simulink model "PD"  (R2020a)
settings: Solver=FixedStepAuto  StartTime=0.0  StopTime=200  RelTol=1e-3  EnableMultiTasking=on
values from neighbouring files (symbols this model uses):
  down = -up    (= -0.0872664625997)    [PD_statespace.m]
  Kx = place(A_d_x,1.1*B_d_x,p_d_x)    [PD_statespace.m]
  Ky = place(A_d_y,1.1*B_d_y,p_d_y)    [PD_statespace.m]
  Ts = 0.02    [PD_statespace.m]
  up = 5*pi/180    (= 0.0872664625997)    [PD_statespace.m]
undefined symbols (not defined in the file or in its folder): A_d_x, A_d_y, B_d_x, B_d_y, C_d_x, C_d_y, DiscIntNeverNeededParam
libraries: raspberrypiBasiclib x6, simulink x4, raspberrypiCommlib x1
settings Model: Creator=hhiastt  LastModifiedBy=hhiastt
settings SolverCC: PositivePriorityOrder=on
settings OptimizationCC: EnhancedBackFolding=on  PassReuseOutputArgsAs=Individual arguments  ZeroExternalMemoryAtStartup=off  ZeroInternalMemoryAtStartup=off  MaxStackSize=64  OptimizeBlockOrder=speed  DifferentSizesBufferReuse=on  OptimizationCustomize=off  EfficientTunableParamExpr=on
settings DebuggingCC: ParameterTunabilityLossMsg=error
settings HardwareCC: ProdBitPerPointer=32  ProdBitPerSizeT=32  ProdBitPerPtrDiffT=32  ProdLargestAtomicInteger=Long  ProdLargestAtomicFloat=Double  ProdWordSize=32  ProdLongLongMode=on  ProdHWDeviceType=ARM Compatible->ARM Cortex
settings RTWCC: SystemTargetFile=ert.tlc  HardwareBoard=Raspberry Pi  TemplateMakefile=ert_default_tmf  Toolchain=GNU GCC Raspberry Pi  BuildConfiguration=Faster Runs
settings CodeAppCC: ForceParamTrailComments=on  IgnoreCustomStorageClasses=off  OperatorAnnotations=on  SimulinkDataObjDesc=on  SFDataObjDesc=on  InsertBlockDesc=on
settings ERTTargetCC: SupportVariableSizeSignals=on

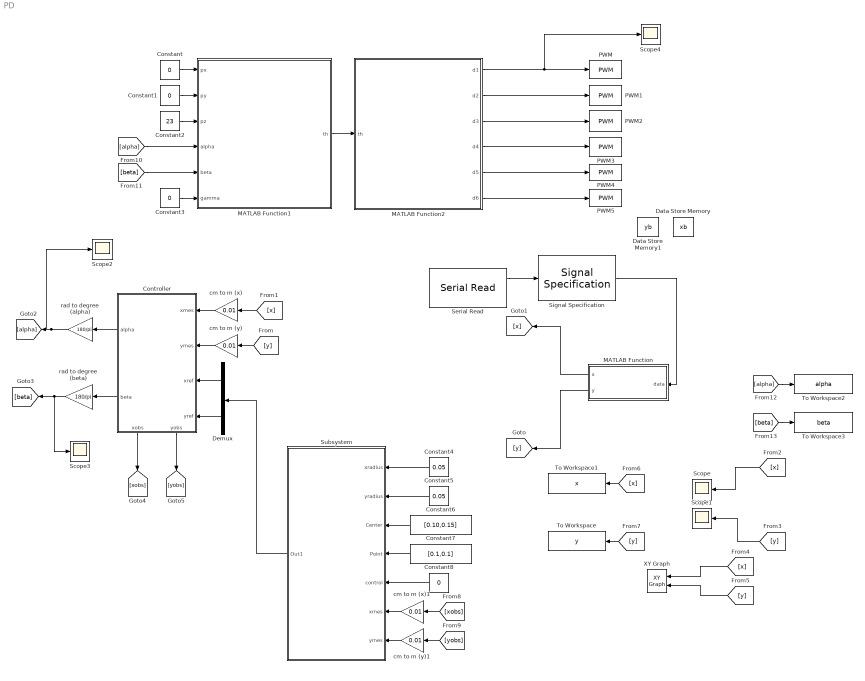
== system PD ==
  Constant{,1,3,8} (4 alike) : Constant  Value=0
  Constant2 : Constant  Value=23
  Constant4 : Constant  Value=0.05
  Constant5 : Constant  Value=0.05
  Constant6 : Constant  Value=[0.10,0.15]
  Constant7 : Constant  Value=[0.1,0.1]
  Controller : Subsystem
      settings: PortSchema="{\"entries\":[{\"content\":{\"sides\":[{\"content\":{\"connectorIds\":[\"In1\",\"In2\",\"In3\",\"In4\"]},\"type\":\"ConnectorPlacement.EquallySpacedRectSide\",\"uuid\":\"b3f4a7cd-8500-437d-beb5-3714d996e55f\"},{\"content\":{\"connectorIds\":[\"Out1\",\"Out2\"],\"side\":\"RIGHT\"},\"type\":\"ConnectorPlacement.EquallySpacedRectSide\",\"uuid\":\"7399a696-fe70-41e1-908f-e26d67b443d7\"},{\"content\":{\"connectorIds\":[],\"side\":\"TOP\"},\"type\":\"ConnectorPlacement.EquallySpacedRectSide\",\"uuid\":\"0bf1a723-c9e2-46e2-b0a4-128eb8cfe212\"},{\"content\":{\"connectorIds\":[\"Out3\",\"Out4\"],\"side\":\"BOTTOM\"},\"type\":\"ConnectorPlacement.EquallySpacedRectSide\",\"uuid\":\"22262538-2ead-478c-9765-503d5c54f33f\"}]},\"type\":\"ConnectorPlacement.EquallySpacedConnector\",\"uuid\":\"64fddb79-6683-4736-8f96-8b1913bbda93\"}],\"packageUris\":[\"http://schema.mathworks.com/mf0/Connector/19700101\"],\"version\":\"1.0\"}"
  Data Store Memory : DataStoreMemory  DataStoreName=xb  ReadBeforeWriteMsg=warning  WriteAfterWriteMsg=warning  WriteAfterReadMsg=warning  ShowAdditionalParam=off  OutDataTypeStr=double
  Data Store Memory1 : DataStoreMemory  DataStoreName=yb  ReadBeforeWriteMsg=warning  WriteAfterWriteMsg=warning  WriteAfterReadMsg=warning  ShowAdditionalParam=off  OutDataTypeStr=double
  Demux : Demux  Outputs=2
  MATLAB Function : MATLAB Function  TreatAsAtomicUnit=on
  MATLAB Function1 : MATLAB Function  TreatAsAtomicUnit=on
  MATLAB Function2 : MATLAB Function  TreatAsAtomicUnit=on
  PWM : raspberrypiBasiclib/PWM  board=Pi 3 Model B+  Pin_=12  Frequency=50  blockPlatform=Raspberry Pi
      settings: SourceProductBaseCode=RASPPI
  PWM1 : raspberrypiBasiclib/PWM  board=Pi 3 Model B+  Pin_=20  Frequency=50  blockPlatform=Raspberry Pi
      settings: SourceProductBaseCode=RASPPI
  PWM2 : raspberrypiBasiclib/PWM  board=Pi 3 Model B+  Pin_=26  Frequency=50  blockPlatform=Raspberry Pi
      settings: SourceProductBaseCode=RASPPI
  PWM3 : raspberrypiBasiclib/PWM  board=Pi 3 Model B+  Pin_=17  Frequency=50  blockPlatform=Raspberry Pi
      settings: SourceProductBaseCode=RASPPI
  PWM4 : raspberrypiBasiclib/PWM  board=Pi 3 Model B+  Pin_=27  Frequency=50  blockPlatform=Raspberry Pi
      settings: SourceProductBaseCode=RASPPI
  PWM5 : raspberrypiBasiclib/PWM  board=Pi 3 Model B+  Pin_=22  Frequency=50  blockPlatform=Raspberry Pi
      settings: SourceProductBaseCode=RASPPI
  Scope{,1..4} (5 alike) : Scope
  Serial Read : raspberrypiCommlib/Serial Read  board=Pi 3 Model B+  SCIModule_=/dev/ttyS0  Baudrate_=19200  Parity=None  StopBits_=1  HardwareFlowControl=None  ByteOrder=LittleEndian  DataLength=10  DataType=uint8  OutputStatus=on  SampleTime=Ts  blockPlatform=RaspberryPi
      settings: SourceProductBaseCode=RASPPI
  Signal Specification : SignalSpecification  OutDataTypeStr=uint8  Dimensions=10  SampleTime=Ts
  Subsystem : Subsystem
  To Workspace : ToWorkspace  VariableName=y  SampleTime=Ts
      settings: Save2DSignal=2-D array (concatenate along first dimension)
  To Workspace1 : ToWorkspace  VariableName=x  SampleTime=Ts
      settings: Save2DSignal=2-D array (concatenate along first dimension)
  To Workspace2 : ToWorkspace  VariableName=alpha  SaveFormat=Timeseries  SampleTime=-1
  To Workspace3 : ToWorkspace  VariableName=beta  SaveFormat=Timeseries  SampleTime=-1
  XY Graph : simulink/Sinks/XY Graph  xmin=0  xmax=20  ymin=0  ymax=30  st=Ts
  cm to m (x) : Gain  Gain=0.01
  cm to m (x)1 : Gain  Gain=0.01
  cm to m (y) : Gain  Gain=0.01
  cm to m (y)1 : Gain  Gain=0.01
  rad to degree (alpha) : Gain  Gain=180/pi
  rad to degree (beta) : Gain  Gain=180/pi
  wires:
  Constant2/1 -> MATLAB Function1/3(pz)
  [x] -> cm to m (x)/1
  MATLAB Function2/5(d5) -> PWM4/1
  Constant8/1 -> Subsystem/5(control)
  rad to degree (beta)/1 -> Scope3/1, [beta]
  [y] -> cm to m (y)/1
  cm to m (x)1/1 -> Subsystem/6(xmes)
  Controller/1(alpha) -> rad to degree (alpha)/1
  Controller/2(beta) -> rad to degree (beta)/1
  Demux/1 -> Controller/3(xref)
  [yobs] -> cm to m (y)1/1
  cm to m (y)/1 -> Controller/2(ymes)
  rad to degree (alpha)/1 -> Scope2/1, [alpha]
  Constant6/1 -> Subsystem/3(Center)
  Constant5/1 -> Subsystem/2(yradius)
  [x] -> To Workspace1/1
  Constant4/1 -> Subsystem/1(xradius)
  [alpha] -> MATLAB Function1/4(alpha)
  [y] -> XY Graph/2
  cm to m (y)1/1 -> Subsystem/7(ymes)
  Constant3/1 -> MATLAB Function1/6(gamma)
  [xobs] -> cm to m (x)1/1
  Constant/1 -> MATLAB Function1/1(px)
  cm to m (x)/1 -> Controller/1(xmes)
  [beta] -> MATLAB Function1/5(beta)
  MATLAB Function2/6(d6) -> PWM5/1
  Signal Specification/1 -> MATLAB Function/1(data)
  MATLAB Function1/1(th) -> MATLAB Function2/1(th)
  [y] -> To Workspace/1
  MATLAB Function/1(x) -> [x]
  MATLAB Function2/2(d2) -> PWM1/1
  [x] -> XY Graph/1
  MATLAB Function2/4(d4) -> PWM3/1
  MATLAB Function2/1(d1) -> Scope4/1, PWM/1
  Constant1/1 -> MATLAB Function1/2(py)
  MATLAB Function/2(y) -> [y]
  Demux/2 -> Controller/4(yref)
  MATLAB Function2/3(d3) -> PWM2/1
  Serial Read/1 -> Signal Specification/1
  Constant7/1 -> Subsystem/4(Point)
  Controller/4(xobs) -> [xobs]
  Controller/3(yobs) -> [yobs]
  Subsystem/1(Out1) -> Demux/1
  [x] -> Scope/1
  [y] -> Scope1/1
  [alpha] -> To Workspace2/1
  [beta] -> To Workspace3/1

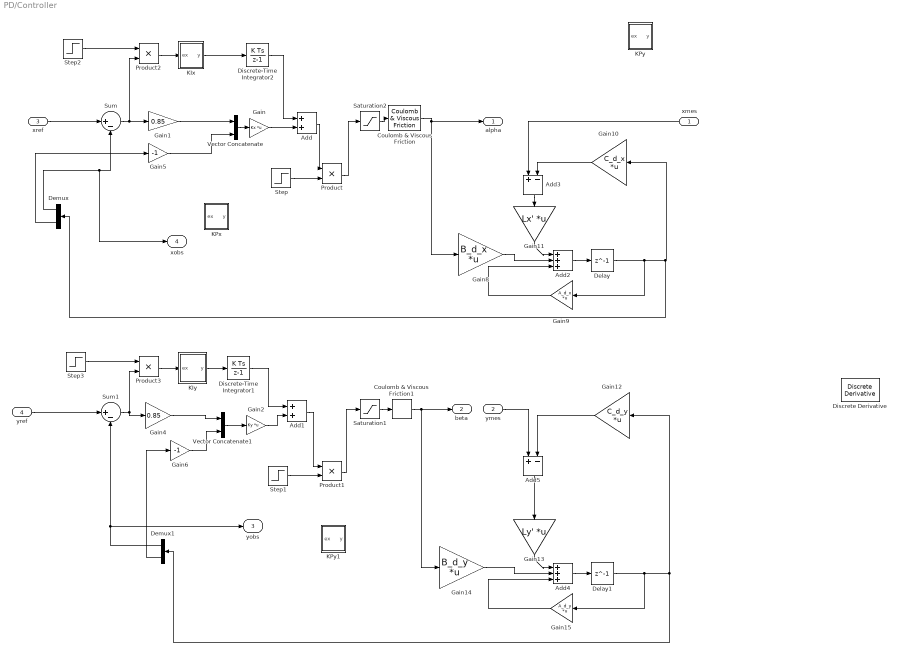
== system PD/Controller ==
  xmes : Inport
  ymes : Inport  Port=2
  xref : Inport  Port=3
  yref : Inport  Port=4
  Add : Sum
  Add1 : Sum
  Add2 : Sum  Inputs=+++
  Add3 : Sum  Inputs=+-
  Add4 : Sum  Inputs=+++
  Add5 : Sum  Inputs=+-
  Coulomb & Viscous Friction : simulink/Discontinuities/Coulomb & Viscous Friction  offset=[0.15*pi/180]  gain=1
  Coulomb & Viscous Friction1 : simulink/Discontinuities/Coulomb & Viscous Friction  offset=[0.15*pi/180]  gain=1
  Delay : Delay  DelayLength=1  SampleTime=Ts
  Delay1 : Delay  DelayLength=1  SampleTime=Ts
  Demux : Demux  Outputs=2
  Demux1 : Demux  Outputs=2
  Discrete Derivative : simulink/Discrete/Discrete Derivative  gainval=1.0  ICPrevScaledInput=0.0  OutMin=[]  OutMax=[]  OutDataType=fixdt(1, 16)  OutScaling=2^-10  DoSatur=off
  Discrete-Time Integrator1 : DiscreteIntegrator  SampleTime=-1  ICPrevOutput=DiscIntNeverNeededParam  ICPrevScaledInput=DiscIntNeverNeededParam
  Discrete-Time Integrator2 : DiscreteIntegrator  SampleTime=-1  ICPrevOutput=DiscIntNeverNeededParam  ICPrevScaledInput=DiscIntNeverNeededParam
  Gain : Gain  Gain=Kx  Multiplication=Matrix(K*u)
  Gain1 : Gain  Gain=0.85
  Gain10 : Gain  Gain=C_d_x  Multiplication=Matrix(K*u)
  Gain11 : Gain  Gain=Lx'  Multiplication=Matrix(K*u)
  Gain12 : Gain  Gain=C_d_y  Multiplication=Matrix(K*u)
  Gain13 : Gain  Gain=Ly'  Multiplication=Matrix(K*u)
  Gain14 : Gain  Gain=B_d_y  Multiplication=Matrix(K*u)
  Gain15 : Gain  Gain=A_d_y  Multiplication=Matrix(K*u)
  Gain2 : Gain  Gain=Ky  Multiplication=Matrix(K*u)
  Gain4 : Gain  Gain=0.85
  Gain5 : Gain  Gain=-1
  Gain6 : Gain  Gain=-1
  Gain8 : Gain  Gain=B_d_x  Multiplication=Matrix(K*u)
  Gain9 : Gain  Gain=A_d_x  Multiplication=Matrix(K*u)
  KIx : MATLAB Function  TreatAsAtomicUnit=on
  KIy : MATLAB Function  TreatAsAtomicUnit=on
  KPx : MATLAB Function  TreatAsAtomicUnit=on
  KPy : MATLAB Function  TreatAsAtomicUnit=on
  KPy1 : MATLAB Function  TreatAsAtomicUnit=on
  Product{,1..3} (4 alike) : Product
  Saturation1 : Saturate  UpperLimit=up  LowerLimit=down
  Saturation2 : Saturate  UpperLimit=up  LowerLimit=down
  Step{,1..3} (4 alike) : Step  Time=4  SampleTime=Ts
  Sum : Sum  Inputs=|+-
  Sum1 : Sum  Inputs=|+-
  Vector Concatenate : Concatenate
  Vector Concatenate1 : Concatenate
  alpha : Outport
  beta : Outport  Port=2
  yobs : Outport  Port=3
  xobs : Outport  Port=4
  wires:
  xref/1 -> Sum/1
  yref/1 -> Sum1/1
  Demux1/2 -> Gain6/1
  Saturation2/1 -> Coulomb & Viscous Friction/1
  xmes/1 -> Add3/1
  Gain9/1 -> Add2/3
  Gain8/1 -> Add2/2
  Gain11/1 -> Add2/1
  Delay/1 -> Demux/1, Gain10/1, Gain9/1
  Add3/1 -> Gain11/1
  Gain10/1 -> Add3/2
  Add2/1 -> Delay/1
  ymes/1 -> Add5/1
  Demux1/1 -> yobs/1, Sum1/2
  Add4/1 -> Delay1/1
  Gain13/1 -> Add4/1
  Add5/1 -> Gain13/1
  Delay1/1 -> Gain15/1, Demux1/1, Gain12/1
  Gain12/1 -> Add5/2
  Gain14/1 -> Add4/2
  Gain15/1 -> Add4/3
  Demux/1 -> xobs/1, Sum/2
  Sum/1 -> Gain1/1, Product2/2
  Demux/2 -> Gain5/1
  Sum1/1 -> Gain4/1, Product3/2
  KIx/1(y) -> Discrete-Time Integrator2/1
  KIy/1(y) -> Discrete-Time Integrator1/1
  Step/1 -> Product/2
  Step1/1 -> Product1/2
  Add/1 -> Product/1
  Product/1 -> Saturation2/1
  Add1/1 -> Product1/1
  Product1/1 -> Saturation1/1
  Step2/1 -> Product2/1
  Product2/1 -> KIx/1(ex)
  Product3/1 -> KIy/1(ex)
  Step3/1 -> Product3/1
  Gain5/1 -> Vector Concatenate/2
  Vector Concatenate/1 -> Gain/1
  Gain/1 -> Add/2
  Vector Concatenate1/1 -> Gain2/1
  Gain6/1 -> Vector Concatenate1/2
  Gain2/1 -> Add1/2
  Gain1/1 -> Vector Concatenate/1
  Gain4/1 -> Vector Concatenate1/1
  Discrete-Time Integrator2/1 -> Add/1
  Discrete-Time Integrator1/1 -> Add1/1
  Coulomb & Viscous Friction/1 -> alpha/1, Gain8/1
  Saturation1/1 -> Coulomb & Viscous Friction1/1
  Coulomb & Viscous Friction1/1 -> beta/1, Gain14/1

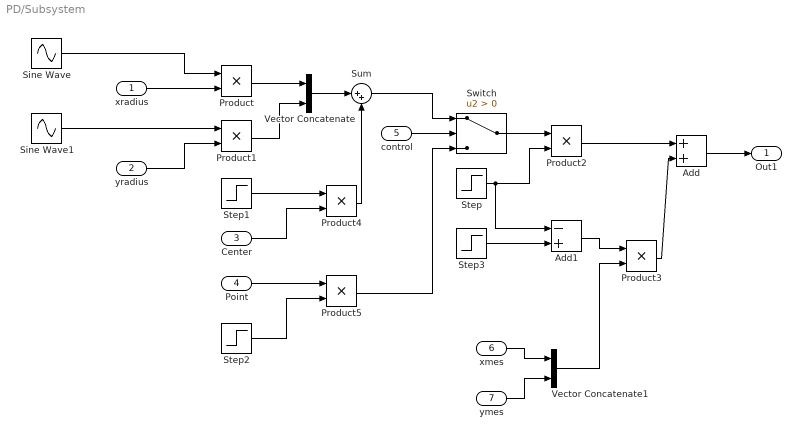
== system PD/Subsystem ==
  xradius : Inport
  yradius : Inport  Port=2
  Center : Inport  Port=3
  Point : Inport  Port=4
  control : Inport  Port=5
  xmes : Inport  Port=6
  ymes : Inport  Port=7
  Add : Sum
  Add1 : Sum  Inputs=-+
  Product{,1..5} (6 alike) : Product
  Sine Wave : Sin  Frequency=0.5  SampleTime=Ts
  Sine Wave1 : Sin  Frequency=0.5  Phase=pi/2  SampleTime=Ts
  Step : Step  Time=4  SampleTime=Ts
  Step1 : Step  Time=0  SampleTime=Ts
  Step2 : Step  Time=0  SampleTime=Ts
  Step3 : Step  Time=0  SampleTime=Ts
  Sum : Sum  Inputs=|++
  Switch : Switch  Criteria=u2 > Threshold
  Vector Concatenate : Concatenate
  Vector Concatenate1 : Concatenate
  Out1 : Outport
  wires:
  Sine Wave/1 -> Product/1
  Sine Wave1/1 -> Product1/1
  xradius/1 -> Product/2
  yradius/1 -> Product1/2
  Product/1 -> Vector Concatenate/1
  Product1/1 -> Vector Concatenate/2
  Vector Concatenate/1 -> Sum/1
  control/1 -> Switch/2
  Sum/1 -> Switch/1
  Product2/1 -> Add/1
  xmes/1 -> Vector Concatenate1/1
  ymes/1 -> Vector Concatenate1/2
  Vector Concatenate1/1 -> Product3/2
  Product3/1 -> Add/2
  Add/1 -> Out1/1
  Switch/1 -> Product2/1
  Step/1 -> Add1/1, Product2/2
  Add1/1 -> Product3/1
  Step1/1 -> Product4/1
  Center/1 -> Product4/2
  Product4/1 -> Sum/2
  Point/1 -> Product5/1
  Product5/1 -> Switch/3
  Step2/1 -> Product5/2
  Step3/1 -> Add1/2

== matlab function PD/MATLAB Function1 ==
  data: px input double size=1; th output double; py input double size=1; pz input double size=1; alpha input double size=1; beta input double size=1; gamma input double size=1
function th = inv_ken_test(px,py,pz,alpha,beta,gamma)
th=zeros(1,6);
l1=3.2;
l2=25.57;
b=26;
d=20;
b1=30;
d1=6;
RA1=[(1/sqrt(12))*(2*b+d);d/2;0];
RA2=[-(1/sqrt(12))*(b-d);(b+d)/2;0];
RA3=[-(1/sqrt(12))*(b+2*d);b/2;0];
RA4=[-(1/sqrt(12))*(b+2*d);-b/2;0];
RA5=[-(1/sqrt(12))*(b-d);-(b+d)/2;0];
RA6=[(1/sqrt(12))*(2*b+d);-d/2;0];
RA=[RA1 RA2 RA3 RA4 RA5 RA6];

RC1=[(1/sqrt(12))*(b1+2*d1);b1/2;0];
RC2=[(1/sqrt(12))*(b1-d1);(b1+d1)/2;0];
RC3=[-(1/sqrt(12))*(2*b1+d1);d1/2;0];
RC4=[-(1/sqrt(12))*(2*b1+d1);-d1/2;0];
RC5=[(1/sqrt(12))*(b1-d1);-(b1+d1)/2;0];
RC6=[(1/sqrt(12))*(b1+2*d1);-b1/2;0];
RC=[RC1 RC2 RC3 RC4 RC5 RC6];

v=[0 0 0 1];
T_base_A1=[rotz(150)*rotx(90) RA1;v];
T_base_A2=[rotz(-30)*rotx(90) RA2;v];
T_base_A3=[rotz(-90)*rotx(90) RA3;v];
T_base_A4=[rotz(90)*rotx(90) RA4;v];
T_base_A5=[rotz(30)*rotx(90) RA5;v];
T_base_A6=[rotz(-150)*rotx(90) RA6;v];

% Computation
R=[rotz(gamma)*roty(beta)*rotx(alpha);0 0 0];
P=[px;py;pz;1];
T=[R P];
RCE=T*[RC;ones(1,6)];
RAE=[RA;ones(1,6)];
L=zeros(1,6);
for i =1:6
    L(i)=sum((RCE(:,i)-RAE(:,i)).^2)^0.5;
end

RA1C1=T_base_A1^(-1)*(RCE(:,1)-RAE(:,1));
RA2C2=T_base_A2^(-1)*(RCE(:,2)-RAE(:,2));
RA3C3=T_base_A3^(-1)*(RCE(:,3)-RAE(:,3));
RA4C4=T_base_A4^(-1)*(RCE(:,4)-RAE(:,4));
RA5C5=T_base_A5^(-1)*(RCE(:,5)-RAE(:,5));
RA6C6=T_base_A6^(-1)*(RCE(:,6)-RAE(:,6));
RAC=[RA1C1 RA2C2 RA3C3 RA4C4 RA5C5 RA6C6];
P1=zeros(1,6);
G1=zeros(1,6);
for i=1:6
    P1(i)=(L(i)^2+l1^2-l2^2)/(2*l1);
end
for i=1:6
    G1(i)=RAC(1,i)^2+RAC(2,i)^2-(P1(i)^2);
end
delta=1;
for i=1:6
    th(i)=atan2d(P1(i)*RAC(2,i)+RAC(1,i)*delta*sqrt(G1(i)), ...
        abs(P1(i)*RAC(1,i)-RAC(2,i)*delta*sqrt(G1(i))));
end

== matlab function PD/MATLAB Function ==
  data: data input; x output; y output; xb data_store_memory; yb data_store_memory
function [x,y] = process_data(data)
global xb
global yb
x=0;y=0;xx=0;yy=0;j=0;data1=zeros(1,4);
data2=zeros(1,4);
for i=1:10
    if(data(i) == 255)
        j=i;
    end
end
if(j <= 6 && j>0)
    data1=data(j+1:j+4);
    data2=cast(data1,'like',zeros(1,4));    
    xx=data2(1)*256+data2(2);
    yy=data2(3)*256+data2(4);
    xx=(xx-floor(floor(xx/128)/2)*128)/2;
    yy=(yy-floor(floor(yy/128)/2)*128)/2;
    x=((xx-20)/470)*22.8;
    y=((yy-7)/490)*30.4;
    xb=x;
    yb=y;
else
    x=xb;
    y=yb;
end
end

== matlab function PD/MATLAB Function2 ==
  data: th input double size=6; d1 output double size=1; d2 output; d3 output; d4 output; d5 output; d6 output
function [d1,d2,d3,d4,d5,d6] =    Angle2duty_test(th)
M1=[0,1.14;10,1.23;20,1.29;30,1.38;40,1.45;50,1.53;60,1.61];
p1=polyfit(M1(:,1),M1(:,2),1);
M2=[0,1.67;10,1.76;20,1.83;30,1.91;40,2];
p2=polyfit(M2(:,1),M2(:,2),1);
M3=[0,1.24;10,1.33;20,1.42;30,1.49;40,1.56;50,1.64];
p3=polyfit(M3(:,1),M3(:,2),1);
M4=[0,1.68;10,1.75;20,1.84;30,1.92;37,1.99];
p4=polyfit(M4(:,1),M4(:,2),1);
M5=[0,1.14;10,1.22;20,1.3;30,1.37;40,1.45;50,1.53];
p5=polyfit(M5(:,1),M5(:,2),1);
M6=[0,1.68;10,1.75;20,1.84;26,1.86];
p6=polyfit(M6(:,1),M6(:,2),1);
d=zeros(1,6);
d1=dot(p1,[th(1),1])/20;
d2=dot(p2,[-th(2),1])/20;
d3=dot(p3,[th(3),1])/20;
d4=dot(p4,[-th(4),1])/20;
d5=dot(p5,[th(5),1])/20;
d6=dot(p6,[-th(6),1])/20;

== matlab function PD/Controller/KIx ==
  data: ex input; y output
function y = fcn(ex)
if((abs(ex)<0.001) )
  y=0;
else
   y=0.04*ex;
end

== matlab function PD/Controller/KPx ==
  data: ex input; y output
function y = fcn(ex)
if((abs(ex)<0.001))
    y=0;
else 
    if((abs(ex)<0.025))
        y=0.8*ex;
    else
        y=ex;
    end
end

== matlab function PD/Controller/KIy ==
  data: y output; ex input
function y = fcn(ex)
if((abs(ex)<0.001))
  y=0;
else
   y=0.04*ex;
end

== matlab function PD/Controller/KPy1 ==
  data: ex input; y output
function y = fcn(ex)
if((abs(ex)<0.001))
    y=0;
else 
    if((abs(ex)<0.025))
        y=0.8*ex;
    else
        y=ex;
    end
end

== matlab function PD/Controller/KPy ==
  data: ex input; y output
function y = fcn(ex)
if((abs(ex)<0.001))
    y=0;
else 
    if((abs(ex)<0.02))
        y=0.8*ex;
    else
        y=ex;
    end
end
